simulink model "segway_lqr"  (R2021b)
settings: Solver=ode45  StartTime=0.0  StopTime=30  MaxStep=0.005  RelTol=1e-4
values from neighbouring files (symbols this model uses):
  A_pitch = [0    1     0     0 ... (first row only)    [vehiculo_autobalanceado_ss.m]
  B_pitch = [0 ... (first row only)    [vehiculo_autobalanceado_ss.m]
  K_lqr = lqr(A_pitch, B_pitch, Q, R)    [Generar_simulink_lqr.m]
settings Model: Creator=crist  LastModifiedBy=crist

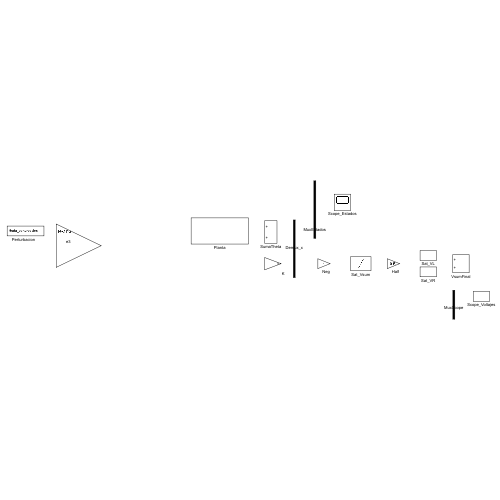
[thumbnail: Simulink's stored preview of the top-level diagram]
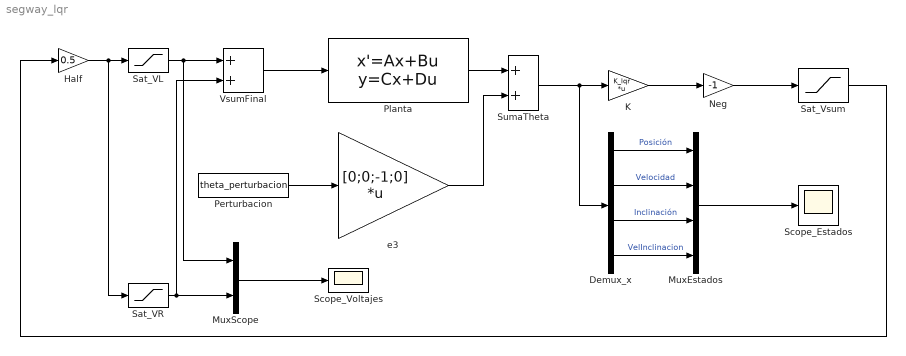
== system segway_lqr ==
  Demux_x : Demux
  Half : Gain  Gain=0.5
  K : Gain  Gain=K_lqr  Multiplication=Matrix(K*u)
  MuxEstados : Mux
  MuxScope : Mux  Inputs=2
  Neg : Gain  Gain=-1
  Perturbacion : FromWorkspace  VariableName=theta_perturbacion
  Planta : StateSpace  A=A_pitch  B=B_pitch  C=eye(4)  D=zeros(4,1)  InitialCondition=[0;0;0;0]
  Sat_VL : Saturate  UpperLimit=24  LowerLimit=-24
  Sat_VR : Saturate  UpperLimit=24  LowerLimit=-24
  Sat_Vsum : Saturate  UpperLimit=48  LowerLimit=-48
  Scope_Estados : Scope
  Scope_Voltajes : Scope
  SumaTheta : Sum
  VsumFinal : Sum
  e3 : Gain  Gain=[0;0;-1;0]  Multiplication=Matrix(K*u)
  wires:
  MuxScope/1 -> Scope_Voltajes/1
  Sat_VR/1 -> VsumFinal/2, MuxScope/2
  VsumFinal/1 -> Planta/1
  Demux_x/1 -> MuxEstados/1  "Posición"
  Demux_x/2 -> MuxEstados/2  "Velocidad"
  Demux_x/4 -> MuxEstados/4  "VelInclinacion"
  Demux_x/3 -> MuxEstados/3  "Inclinación"
  MuxEstados/1 -> Scope_Estados/1
  Sat_Vsum/1 -> Half/1
  Neg/1 -> Sat_Vsum/1
  K/1 -> Neg/1
  e3/1 -> SumaTheta/2
  Planta/1 -> SumaTheta/1
  Perturbacion/1 -> e3/1
  Sat_VL/1 -> VsumFinal/1, MuxScope/1
  Half/1 -> Sat_VL/1, Sat_VR/1
  SumaTheta/1 -> Demux_x/1, K/1
